simulink model "FourCellImplementation"  (R2021b)
settings: Solver=VariableStepAuto  StartTime=0.0  StopTime=1500  RelTol=1e-3
libraries: spsVoltageMeasurementLib x6, spsDiodeLib x4, spsSeriesRLCBranchLib x4, spsLinearTransformerLib x2, spsGroundLib x1, spsMosfetLib x1, spspowerguiLib x1
settings Model: Creator=HP  LastModifiedBy=rajra
settings SolverCC: AlgebraicLoopSolver=TrustRegion
settings DebuggingCC: SFMachineParentedDataDiag=warning

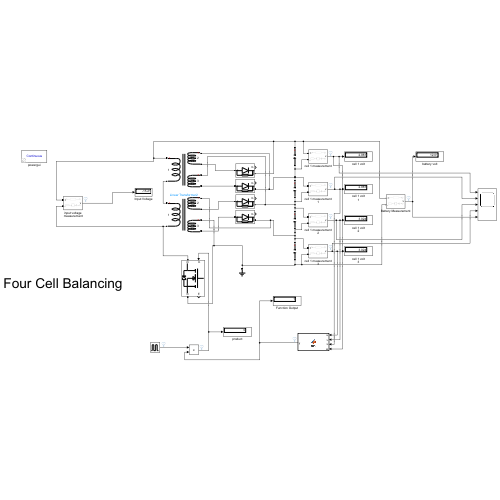
[thumbnail: Simulink's stored preview of the top-level diagram]
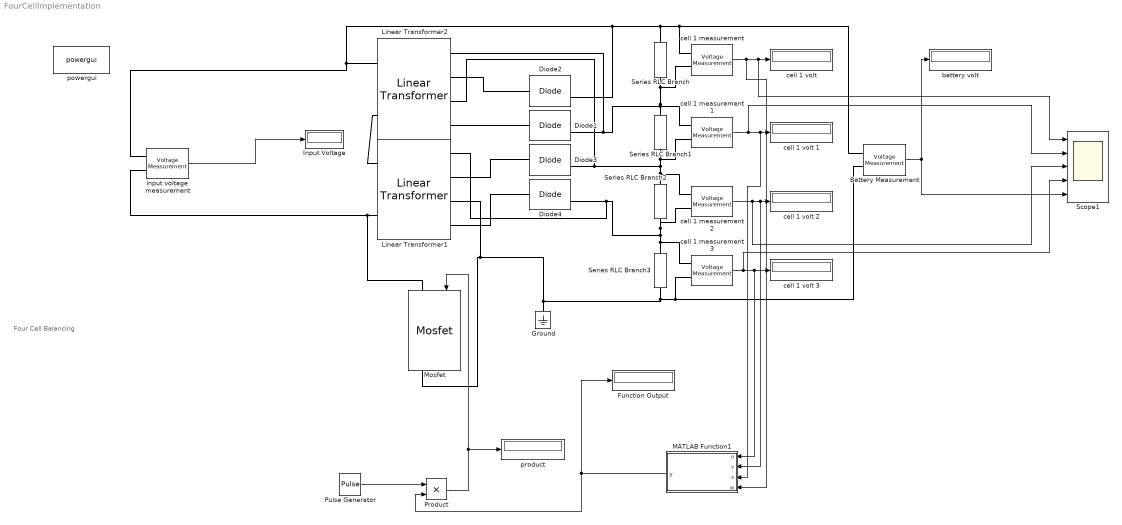
== system FourCellImplementation ==
  note: Four Cell Balancing
  "Battery Measurement " : spsVoltageMeasurementLib/Voltage Measurement  PhasorSimulation=off  OutputType=Complex  PSBequivalent=0
  Diode{1..4} (4 alike) : spsDiodeLib/Diode  Ron=0.001  Lon=0  Vf=0.8  IC=0  UseSnubber=0  Rs=500  Cs=250e-9  Measurements=on
  Function Output : Display
  Ground : spsGroundLib/Ground  LConnTagsString=a
  Input Voltage : Display
  Linear Transformer1 : spsLinearTransformerLib/Linear Transformer  UNITS=SI  NominalPower=[100 55000]  winding1=[10 0.02 45e-6]  winding2=[5 0.02 288e-6]  ThreeWindings=on  winding3=[5 0.02 288e-6]  RmLm=[1.0805e+06 2866]  Measurements=None  DataType=on
  Linear Transformer2 : spsLinearTransformerLib/Linear Transformer  UNITS=SI  NominalPower=[100 55000]  winding1=[10 0.02 45e-6]  winding2=[5 0.02 288e-6]  ThreeWindings=on  winding3=[5 0.02 288e-6]  RmLm=[1.0805e+06 2866]  Measurements=None  DataType=on
  MATLAB Function1 : MATLAB Function  TreatAsAtomicUnit=on
  Mosfet : spsMosfetLib/Mosfet  Ron=1.5  Lon=0  Rd=2  Vfd=0  IC=0  Rs=1500  Cs=288e-7  Measurements=on
  Product : Product
  Pulse Generator : DiscretePulseGenerator  PulseType=Time based  Period=10  PulseWidth=50
  Scope1 : Scope  NumInputPorts=5
  Series RLC Branch : spsSeriesRLCBranchLib/Series RLC Branch  LConnTagsString=__new0  RConnTagsString=__new0  BranchType=C  Resistance=1  Inductance=1e-3  SetiL0=off  InitialCurrent=0  Capacitance=5  Setx0=on  InitialVoltage=2.8  Measurements=None
  Series RLC Branch1 : spsSeriesRLCBranchLib/Series RLC Branch  LConnTagsString=__new0  RConnTagsString=__new0  BranchType=C  Resistance=1  Inductance=1e-3  SetiL0=off  InitialCurrent=0  Capacitance=5  Setx0=on  InitialVoltage=3.3  Measurements=None
  Series RLC Branch2 : spsSeriesRLCBranchLib/Series RLC Branch  LConnTagsString=__new0  RConnTagsString=__new0  BranchType=C  Resistance=1  Inductance=1e-3  SetiL0=off  InitialCurrent=0  Capacitance=5  Setx0=on  InitialVoltage=2.9  Measurements=None
  Series RLC Branch3 : spsSeriesRLCBranchLib/Series RLC Branch  LConnTagsString=__new0  RConnTagsString=__new0  BranchType=C  Resistance=1  Inductance=1e-3  SetiL0=off  InitialCurrent=0  Capacitance=5  Setx0=on  InitialVoltage=3.3  Measurements=None
  "battery volt " : Display
  cell 1 measurement {,1..3} (4 alike) : spsVoltageMeasurementLib/Voltage Measurement  PhasorSimulation=off  OutputType=Complex  PSBequivalent=0
  cell 1 volt {,1..3} (4 alike) : Display
  "input voltage measurement " : spsVoltageMeasurementLib/Voltage Measurement  PhasorSimulation=off  OutputType=Complex  PSBequivalent=0
  powergui : spspowerguiLib/powergui  Priority=1  SimulationMode=Continuous  SampleTime=50e-6  frequency=60  Iterations=50  frequencyindice=0  Pbase=100e6  ErrMax=1e-4  UnitsV=kV  UnitsW=MW  buscounter=0  FunctionMessages=off  echomessages=off  EnableUseOfTLC=off  CurrentSourceSwitches=off  DisableSnubberDevices=off  DisableRonSwitches=off  DisableVfSwitches=off  DisplayEquations=off  AutomaticDiscreteSolvers=off  SolverType=Tustin/Backward Euler (TBE)  Interpol=off  ExternalGateDelay=off  methode=off  Ts=100  x0status=blocks  SPID=on  SwTol=0  HookPort=off  NonlinearTolerance=1e-4  nMaxIteration=100  ContinueOnMaxIteration=off  RestoreLinks=warning  ResistiveCurrentMeasurement=off  Frange=[0:2:500]  Ylog=off  Xlog=on  ShowGrid=off  save=off  variable=ZData  structure=0  ZoomFFT=off  StartTime=0.0  cycles=1  DisplayStyle=1  fundamental=60  FreqAxis=off  MaxFrequency=1000  frequencyindicesteady=1  RmsSteady=1  display=off
  "product " : Display
  wires:
  "input voltage measurement "/1 -> Input Voltage/1
  Pulse Generator/1 -> Product/1
  Product/1 -> "product "/1, Mosfet/1
  MATLAB Function1/1(y) -> Product/2, Function Output/1
  "cell 1 measurement "/1 -> MATLAB Function1/4(w), Scope1/1, "cell 1 volt "/1
  cell 1 measurement 1/1 -> Scope1/2, MATLAB Function1/3(x), cell 1 volt 1/1
  cell 1 measurement 2/1 -> Scope1/3, MATLAB Function1/2(v), cell 1 volt 2/1
  "Battery Measurement "/1 -> "battery volt "/1, Scope1/5
  cell 1 measurement 3/1 -> Scope1/4, MATLAB Function1/1(u), cell 1 volt 3/1
  connections:
  Series RLC Branch/LConn1 -- "Battery Measurement "/LConn1 -- "cell 1 measurement "/LConn1 -- "input voltage measurement "/LConn1 -- Linear Transformer2/LConn1 -- Diode2/RConn1
  "input voltage measurement "/LConn2 -- Mosfet/LConn1 -- Linear Transformer1/LConn2
  Series RLC Branch3/LConn1 -- cell 1 measurement 3/LConn1 -- Linear Transformer1/RConn1 -- Diode4/RConn1 -- cell 1 measurement 2/LConn2 -- Series RLC Branch2/RConn1
  Series RLC Branch1/RConn1 -- cell 1 measurement 1/LConn2 -- Linear Transformer2/RConn3 -- Diode3/RConn1 -- cell 1 measurement 2/LConn1 -- Series RLC Branch2/LConn1
  Series RLC Branch1/LConn1 -- cell 1 measurement 1/LConn1 -- Linear Transformer2/RConn1 -- Diode1/RConn1 -- "cell 1 measurement "/LConn2 -- Series RLC Branch/RConn1
  Series RLC Branch3/RConn1 -- "Battery Measurement "/LConn2 -- cell 1 measurement 3/LConn2 -- Mosfet/RConn1 -- Linear Transformer1/RConn3 -- Ground/LConn1
  Diode2/LConn1 -- Linear Transformer2/RConn2
  Diode1/LConn1 -- Linear Transformer2/RConn4
  Linear Transformer1/RConn2 -- Diode3/LConn1
  Linear Transformer1/RConn4 -- Diode4/LConn1
  Linear Transformer1/LConn1 -- Linear Transformer2/LConn2

== matlab function FourCellImplementation/MATLAB Function1 ==
  data: u input; y output; v input; x input; w input
function y = fcn(u,v,x,w)
if(u <= v && u >= v &&  v<= w && v>= w && v <= x && v >= x)
    y = 0;
else 
    y = 1;
end
